simulink model "aeropropmodel"  (Simulink 3.00)
settings: Solver=ode45  StartTime=0.0  StopTime=10.0  RelTol=1e-3
libraries: simulink3 x1, fdclib2 x1, fdclib3 x1
settings Model: LastModifiedBy=Dutchroll

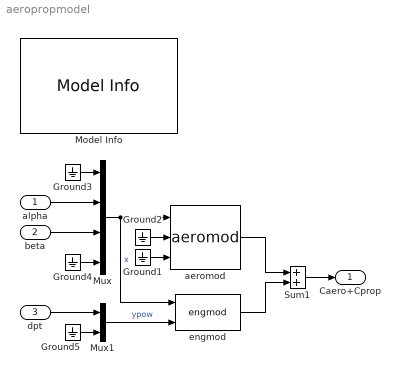
== system aeropropmodel ==
  alpha : Inport  Port=1  PortWidth=-1  SampleTime=-1  DataType=auto
      settings: SignalType=auto
  beta : Inport  Port=2  PortWidth=-1  SampleTime=-1  DataType=auto
      settings: SignalType=auto
  dpt : Inport  Port=3  PortWidth=-1  SampleTime=-1  DataType=auto
      settings: SignalType=auto
  Ground{1..5} (5 alike) : Ground
  Model Info : simulink3/Signals & Systems/Model Info  InitialBlockCM=none  BlockCM=none  Frame=on  DisplayStringWithTags=|  HorizontalTextAlignment=Center  LeftAlignmentValue=0.5  SourceBlockDiagram=aeropropmodel  TagMaxNumber=20
      | Test system to validate the 
      | aerodynamic and propulsive 
      | forces and moments models.
      | Used by PROPCOEFF.M.
      | 
      | M.O. Rauw, March 2004
  Mux : Mux  Inputs=[1 1 1 9]
  Mux1 : Mux  Inputs=2
  Sum1 : Sum  Inputs=++  SaturateOnIntegerOverflow=on
  aeromod : fdclib2/aeromod
  engmod : fdclib3/engmod
  Caero+Cprop : Outport  Port=1
  wires:
  aeromod/1 -> Sum1/1
  engmod/1 -> Sum1/2
  Sum1/1 -> Caero+Cprop/1
  Ground1/1 -> aeromod/3
  Ground2/1 -> aeromod/2
  Mux/1 -> aeromod/1, engmod/1  "x"
  alpha/1 -> Mux/2
  beta/1 -> Mux/3
  Ground3/1 -> Mux/1
  Ground4/1 -> Mux/4
  Mux1/1 -> engmod/2  "ypow"
  Ground5/1 -> Mux1/2
  dpt/1 -> Mux1/1
